simulink model "control_pos_3dof_sinMI"  (R2023b)
settings: Solver=ode5  StartTime=0.0  StopTime=tsim  FixedStep=tstep  RelTol=1e-3
undefined symbols (not defined in the file): a0, a1, robot_params, t_qeq_init, t_tr_init, tau_L
(part 2 of 2)

== matlab function control_pos_3dof_sinMI/Modelo robot manipulador (Dinámica directa)/Modelo dinámico ==
  data: robot_params input; robot_din output Bus: robot_din_bus size=1; q input size=[3,1]; dq input size=[3,1]
function robot_din = fcn(robot_params,q,dq)

%d1 = robot_params.d(1);
l2 = robot_params.l(2);
lc2 = robot_params.lc(2);
%l3 = robot_params.l(3);
lc3 = robot_params.lc(3);

%m1 = robot_params.m(1);
m2 = robot_params.m(2);
m3 = robot_params.m(3);

Iz1 = robot_params.I(1,3);
Iy2 = robot_params.I(2,2);
Iz2 = robot_params.I(2,3);
Iy3 = robot_params.I(3,2);
Iz3 = robot_params.I(3,3);

g = 9.81;

q1 = q(1);
q2 = q(2);
q3 = q(3);

dq1 = dq(1);
dq2 = dq(2);
dq3 = dq(3);

D = zeros(3,3);

D(1,1) = Iz1 + Iz2 + Iz3 + (m2/2)*lc2^2*(1+cos(2*q2)) ...
       + (m3/2)*(l2^2*(1+cos(2*q2)) + 2*l2*lc3*(cos(2*q2+q3)+cos(q3)) ...
       + lc3^2*(1+cos(2*q2+2*q3)));

D(2,2) = Iy2 + Iy3 + m2*lc2^2 + m3*(l2^2 + 2*l2*lc3*cos(q3) + lc3^2);
D(2,3) = Iy3 + m3*(l2*lc3*cos(q3) + lc3^2);

D(3,2) = Iy3 + m3*(l2*lc3*cos(q3) + lc3^2);
D(3,3) = Iy3 + m3*lc3^2;

C = zeros(3,3);

C(1,2) = - ((m2*lc2^2*sin(2*q2)) ...
         + m3*(l2^2*sin(2*q2) + 2*l2*lc3*sin(2*q2+q3) ...
         + lc3^2*sin(2*q2+2*q3)))*dq1;
C(1,3) = - m3*(l2*lc3*(sin(2*q2+q3)+sin(q3)) ...
         + lc3^2*(sin(2*q2+2*q3)))*dq1;

C(2,1) =   ((m2/2)*(lc2^2*sin(2*q2)) ...
         + (m3/2)*(l2^2*sin(2*q2) + 2*l2*lc3*sin(2*q2+q3) ...
         + lc3^2*sin(2*q2+2*q3)))*dq1;
C(2,2) = - 2*m3*l2*lc3*sin(q3)*dq3;
C(2,3) = - m3*l2*lc3*sin(q3)*dq3;

C(3,1) =   (m3/2)*(l2*lc3*(sin(2*q2+q3) + sin(q3)) ...
         + lc3^2*sin(2*q2+2*q3))*dq1;
C(3,2) =   m3*l2*lc3*sin(q3)*dq2;

G = zeros(3,1);

G(2,1) = m2*lc2*cos(q2) + m3*(l2*cos(q2) + lc3*cos(q2+q3));
G(3,1) = m3*lc3*cos(q2+q3);


robot_din = struct('D',D,'C',C,'G',G,'g',9.81);

%busInfo = Simulink.Bus.createObject(robot_dyn);

== matlab function control_pos_3dof_sinMI/q to xyz (robot)/Cinemática directa ==
  data: robot_params input; p output size=[3,3]; q input size=[3,1]
function p  = fcn(robot_params,q)

d1 = robot_params.d(1);
l2 = robot_params.l(2);
l3 = robot_params.l(3);

q1 = q(1);
q2 = q(2);
q3 = q(3);

p1 = [0;0;d1];

p2 = [l2*cos(q1)*cos(q2);
      l2*sin(q1)*cos(q2);
      d1+l2*sin(q2)];

p3 = [cos(q1)*(l2*cos(q2)+l3*cos(q2+q3));
      sin(q1)*(l2*cos(q2)+l3*cos(q2+q3));
      d1+l2*sin(q2)+l3*sin(q2+q3)];

p = [p1,p2,p3];

== matlab function control_pos_3dof_sinMI/q to xyz (referencia)/ddq to ddp ==
  data: dJP input size=[3,3]; ddp output size=[3,1]; ddq input size=[3,1]
function ddp = fcn(dJP,ddq)

ddp = dJP*ddq;

== matlab function control_pos_3dof_sinMI/q to xyz (referencia)/dq to dp ==
  data: JP input size=[3,3]; dp output size=[3,1]; dq input size=[3,1]
function dp = fcn(JP,dq)

dp = JP*dq;

== matlab function control_pos_3dof_sinMI/q to xyz (robot)/Jacobiano ==
  data: robot_params input; JP output size=[3,3]; q input size=[3,1]
function JP = fcn(robot_params,q)

l2 = robot_params.l(2);
l3 = robot_params.l(3);

q1 = q(1);
q2 = q(2);
q3 = q(3);

JP = zeros(3,3);

JP(1,1) = -sin(q1)*(l2*cos(q2) + l3*cos(q2 + q3));
JP(1,2) = -cos(q1)*(l2*sin(q2) + l3*sin(q2 + q3));
JP(1,3) = -l3*cos(q1)*sin(q2 + q3);

JP(2,1) =  cos(q1)*(l2*cos(q2) + l3*cos(q2 + q3));
JP(2,2) = -sin(q1)*(l2*sin(q2) + l3*sin(q2 + q3));
JP(2,3) = -l3*sin(q1)*sin(q2 + q3);

JP(3,2) = l2*cos(q2) + l3*cos(q2 + q3);
JP(3,3) = l3*cos(q2 + q3);

== matlab function control_pos_3dof_sinMI/q to xyz (robot)/ddq to ddp ==
  data: dJP input size=[3,3]; ddp output size=[3,1]; ddq input size=[3,1]
function ddp = fcn(dJP,ddq)

ddp = dJP*ddq;

== matlab function control_pos_3dof_sinMI/q to xyz (robot)/derivada Jacobiano ==
  data: robot_params input; q input size=[3,1]; dJP output size=[3,3]; dq input size=[3,1]
function dJP = dJP(robot_params,q,dq)

l2 = robot_params.l(2);
l3 = robot_params.l(3);

dq1 = dq(1);
dq2 = dq(2);
dq3 = dq(3);


q1 = q(1);
q2 = q(2);
q3 = q(3);

dJP = zeros(3,3);

dJP(1,1) = - cos(q1)*(l2*cos(q2) + l3*cos(q2 + q3))*dq1 + sin(q1)*(l2*sin(q2) + l3*sin(q2 + q3))*dq2 + l3*sin(q1)*sin(q2 + q3)*dq3;
dJP(1,2) =   sin(q1)*(l2*sin(q2) + l3*sin(q2 + q3))*dq1 - cos(q1)*(l2*cos(q2) + l3*cos(q2 + q3))*dq2 - l3*cos(q1)*cos(q2 + q3)*dq3;
dJP(1,3) =   l3*sin(q1)*sin(q2 + q3)*dq1 - l3*cos(q1)*cos(q2 + q3)*dq2 - l3*cos(q1)*cos(q2 + q3)*dq3;

dJP(2,1) = - sin(q1)*(l2*cos(q2) + l3*cos(q2 + q3))*dq1 - cos(q1)*(l2*sin(q2) + l3*sin(q2 + q3))*dq2 - l3*cos(q1)*sin(q2 + q3)*dq3;
dJP(2,2) = - cos(q1)*(l2*sin(q2) + l3*sin(q2 + q3))*dq1 - sin(q1)*(l2*cos(q2) + l3*cos(q2 + q3))*dq2 - l3*sin(q1)*cos(q2 + q3)*dq3;
dJP(2,3) = - l3*cos(q1)*sin(q2 + q3)*dq1 - l3*sin(q1)*cos(q2 + q3)*dq2 - l3*sin(q1)*cos(q2 + q3)*dq3;

dJP(3,1) = 0;
dJP(3,2) = - (l2*sin(q2) + l3*sin(q2 + q3))*dq2 - l3*sin(q2 + q3)*dq3;
dJP(3,3) = - l3*sin(q2 + q3)*(dq2 + dq3);

== matlab function control_pos_3dof_sinMI/Modelo robot manipulador (Dinámica directa)/Dinámica directa ==
  data: robot_din input; ddq output size=[3,1]; dq input size=[3,1]; tau_R input size=[3,1]; tau_L input size=[3,1]
function ddq = fcn(robot_din,dq,tau_R,tau_L)

D = robot_din.D;
C = robot_din.C;
G = robot_din.G;
g = robot_din.g;

ddq = D^-1*(-C*dq-G*g+(tau_R-tau_L));

== matlab function control_pos_3dof_sinMI/xyz to q (referencia)/xyz to q (referencia) ==
  data: robot_params input; q output size=[3,1]; r input size=[3,1]; dr input size=[3,1]; ddr input size=[3,1]; dq output size=[3,1]; ddq output size=[3,1]
function [q,dq,ddq] = fcn(robot_params,r,dr,ddr)

d1 = robot_params.d(1);
l2 = robot_params.l(2);
l3 = robot_params.l(3);

Xr = r(1);
Yr = r(2);
Zr = r(3);


c3 = (Xr^2+Yr^2+(Zr-d1)^2-l2^2-l3^2)/(2*l2*l3);

q1 = atan2(Yr,Xr);
q2 = atan2(Zr-d1,sqrt(Xr^2+Yr^2)) - atan2(-l3*sqrt(1-c3^2),l2+l3*c3);
q3 = atan2(-sqrt(1-c3^2),c3);

q = [q1;q2;q3];

JPinv = zeros(3,3);
JPinv(1,1) = -sin(q1)/(l2*cos(q2) + l3*cos(q2 + q3));
JPinv(1,2) = cos(q1)/(l2*cos(q2) + l3*cos(q2 + q3));

JPinv(2,1) = cos(q1)*cos(q2 + q3)/(l2*sin(q3));
JPinv(2,2) = sin(q1)*cos(q2 + q3)/(l2*sin(q3));
JPinv(2,3) = sin(q2 + q3)/(l2*sin(q3));

JPinv(3,1) = -(cos(q1)*(l2*cos(q2) + l3*cos(q2 + q3)))/(l2*l3*sin(q3));
JPinv(3,2) = -(sin(q1)*(l2*cos(q2) + l3*cos(q2 + q3)))/(l2*l3*sin(q3));
JPinv(3,3) = -(l2*sin(q2) + l3*sin(q2 + q3))/(l2*l3*sin(q3));

dq = JPinv*dr;

dq1 = dq(1);
dq2 = dq(2);
dq3 = dq(3);


dJ = zeros(3,3);

dJ(1,1) = - cos(q1)*(l2*cos(q2) + l3*cos(q2 + q3))*dq1 + sin(q1)*(l2*sin(q2) + l3*sin(q2 + q3))*dq2 + l3*sin(q1)*sin(q2 + q3)*dq3;
dJ(1,2) =   sin(q1)*(l2*sin(q2) + l3*sin(q2 + q3))*dq1 - cos(q1)*(l2*cos(q2) + l3*cos(q2 + q3))*dq2 - l3*cos(q1)*cos(q2 + q3)*dq3;
dJ(1,3) =   l3*sin(q1)*sin(q2 + q3)*dq1 - l3*cos(q1)*cos(q2 + q3)*dq2 - l3*cos(q1)*cos(q2 + q3)*dq3;

dJ(2,1) = - sin(q1)*(l2*cos(q2) + l3*cos(q2 + q3))*dq1 - cos(q1)*(l2*sin(q2) + l3*sin(q2 + q3))*dq2 - l3*cos(q1)*sin(q2 + q3)*dq3;
dJ(2,2) = - cos(q1)*(l2*sin(q2) + l3*sin(q2 + q3))*dq1 - sin(q1)*(l2*cos(q2) + l3*cos(q2 + q3))*dq2 - l3*sin(q1)*cos(q2 + q3)*dq3;
dJ(2,3) = - l3*cos(q1)*sin(q2 + q3)*dq1 - l3*sin(q1)*cos(q2 + q3)*dq2 - l3*sin(q1)*cos(q2 + q3)*dq3;

dJ(3,1) = 0;
dJ(3,2) = - (l2*sin(q2) + l3*sin(q2 + q3))*dq2 - l3*sin(q2 + q3)*dq3;
dJ(3,3) = - l3*sin(q2 + q3)*(dq2 + dq3);

ddq = JPinv*(ddr - dJ*dq);

== matlab function control_pos_3dof_sinMI/q to xyz (robot)/dq to dp ==
  data: JP input size=[3,3]; dp output size=[3,1]; dq input size=[3,1]
function dp = fcn(JP,dq)

dp = JP*dq;

== matlab function control_pos_3dof_sinMI/q to xyz (robot)/q to xyz (referencia) ==
  data: robot_params input; p output size=[3,3]; q input size=[3,1]; dq input size=[3,1]; ddq input size=[3,1]; dp output size=[3,1]; ddp output size=[3,1]
function [p,dp,ddp] = fcn(robot_params,q,dq,ddq)

d1 = robot_params.d(1);
l2 = robot_params.l(2);
l3 = robot_params.l(3);

q1 = q(1);
q2 = q(2);
q3 = q(3);

p1 = [0;0;d1];

p2 = [l2*cos(q1)*cos(q2);
      l2*sin(q1)*cos(q2);
      d1+l2*sin(q2)];

p3 = [cos(q1)*(l2*cos(q2)+l3*cos(q2+q3));
      sin(q1)*(l2*cos(q2)+l3*cos(q2+q3));
      d1+l2*sin(q2)+l3*sin(q2+q3)];

p = [p1,p2,p3];

JP = zeros(3,3);

JP(1,1) = -sin(q1)*(l2*cos(q2) + l3*cos(q2 + q3));
JP(1,2) = -cos(q1)*(l2*sin(q2) + l3*sin(q2 + q3));
JP(1,3) = -l3*cos(q1)*sin(q2 + q3);

JP(2,1) =  cos(q1)*(l2*cos(q2) + l3*cos(q2 + q3));
JP(2,2) = -sin(q1)*(l2*sin(q2) + l3*sin(q2 + q3));
JP(2,3) = -l3*sin(q1)*sin(q2 + q3);

JP(3,2) = l2*cos(q2) + l3*cos(q2 + q3);
JP(3,3) = l3*cos(q2 + q3);

dp = JP*dq;
dq1 = dq(1);
dq2 = dq(2);
dq3 = dq(3);

dJ = zeros(3,3);

dJ(1,1) = - cos(q1)*(l2*cos(q2) + l3*cos(q2 + q3))*dq1 + sin(q1)*(l2*sin(q2) + l3*sin(q2 + q3))*dq2 + l3*sin(q1)*sin(q2 + q3)*dq3;
dJ(1,2) =   sin(q1)*(l2*sin(q2) + l3*sin(q2 + q3))*dq1 - cos(q1)*(l2*cos(q2) + l3*cos(q2 + q3))*dq2 - l3*cos(q1)*cos(q2 + q3)*dq3;
dJ(1,3) =   l3*sin(q1)*sin(q2 + q3)*dq1 - l3*cos(q1)*cos(q2 + q3)*dq2 - l3*cos(q1)*cos(q2 + q3)*dq3;

dJ(2,1) = - sin(q1)*(l2*cos(q2) + l3*cos(q2 + q3))*dq1 - cos(q1)*(l2*sin(q2) + l3*sin(q2 + q3))*dq2 - l3*cos(q1)*sin(q2 + q3)*dq3;
dJ(2,2) = - cos(q1)*(l2*sin(q2) + l3*sin(q2 + q3))*dq1 - sin(q1)*(l2*cos(q2) + l3*cos(q2 + q3))*dq2 - l3*sin(q1)*cos(q2 + q3)*dq3;
dJ(2,3) = - l3*cos(q1)*sin(q2 + q3)*dq1 - l3*sin(q1)*cos(q2 + q3)*dq2 - l3*sin(q1)*cos(q2 + q3)*dq3;

dJ(3,1) = 0;
dJ(3,2) = - (l2*sin(q2) + l3*sin(q2 + q3))*dq2 - l3*sin(q2 + q3)*dq3;
dJ(3,3) = - l3*sin(q2 + q3)*(dq2 + dq3);

ddp = dJ*ddq;

== matlab function control_pos_3dof_sinMI/Controlador/Controlador ==
  data: robot_din input; tau_R output size=[3,1]; A0 input size=[3,1]; A1 input size=[3,1]; q_ref input size=[3,1]; dq_ref input size=[3,1]; ddq_ref input size=[3,1]; q input size=[3,1]; dq input size=[3,1]
function tau_R = fcn(robot_din,A0,A1,q_ref,dq_ref,ddq_ref,q,dq)

D = robot_din.D;
C = robot_din.C;
G = robot_din.G;
g = robot_din.g;

tau_R = D*(ddq_ref+A1.*dq_ref+A0.*q_ref-A1.*dq-A0.*q)+(C*dq+G*g);

== matlab function control_pos_3dof_sinMI/Inicializar posición de robot manipulador/dq_init/q1/Polinomio 7mo orden dq ==
  data: t input; q0 input; qpol output; vpol output; apol output; jpol output; q1 input; t0 input; t1 input
function [qpol,vpol,apol,jpol] = fcn(t,q0,q1,t0,t1)


% t,q0,q1,v0,v1,ac0,ac1,j0,j1,t0,t1)
%Trayectoria de referencia

% q0 = 0;
% q1 = 0;

v0 = 0;
v1 = 0;

ac0 = 0;
ac1 = 0;

j0 = 0;
j1 = 0;

% t0 = 0;
% t1 = pi/4;

% Coeficientes de un polinomio de 7mo grado

h = q1 - q0;
T = t1 - t0;

a = zeros(7+1,1);

a(1) = q0;
a(2) = v0;
a(3) = ac0/2;
a(4) = j0/6;
a(5) = (210*h-T*((30*ac0-15*ac1)*T+(4*j0+j1)*T^2+120*v0+90*v1))/(6*T^4);
a(6) = (-168*h-T*((20*ac0-14*ac1)*T+(2*j0+j1)*T^2+90*v0+78*v1))/(2*T^5);
a(7) = (420*h-T*((45*ac0-39*ac1)*T+(4*j0+3*j1)*T^2+216*v0+204*v1))/(6*T^6);
a(8) = (-120*h-T*((12*ac0-12*ac1)*T+(j0+j1)*T^2+60*v0+60*v1))/(6*T^7);

qa = flip(a')';
va = polyder(qa')';
aa = polyder(va')';
ja = polyder(aa')';


if t>=t0 && t<t1
    qpol = polyval(qa,t-t0);
    vpol = polyval(va,t-t0);
    apol = polyval(aa,t-t0);
    jpol = polyval(ja,t-t0);
elseif t>=t1
    qpol = polyval(qa,T);
    vpol = polyval(va,T);
    apol = polyval(aa,T);
    jpol = polyval(ja,T);
else
    qpol = q0;
    vpol = v0;
    apol = ac0;
    jpol = j0;
end

== matlab function control_pos_3dof_sinMI/Inicializar posición de robot manipulador/dq_init/q2/Polinomio 7mo orden dq ==
  data: t input; q0 input; qpol output; vpol output; apol output; jpol output; q1 input; t0 input; t1 input
function [qpol,vpol,apol,jpol] = fcn(t,q0,q1,t0,t1)


% t,q0,q1,v0,v1,ac0,ac1,j0,j1,t0,t1)
%Trayectoria de referencia

% q0 = 0;
% q1 = 0;

v0 = 0;
v1 = 0;

ac0 = 0;
ac1 = 0;

j0 = 0;
j1 = 0;

% t0 = 0;
% t1 = pi/4;

% Coeficientes de un polinomio de 7mo grado

h = q1 - q0;
T = t1 - t0;

a = zeros(7+1,1);

a(1) = q0;
a(2) = v0;
a(3) = ac0/2;
a(4) = j0/6;
a(5) = (210*h-T*((30*ac0-15*ac1)*T+(4*j0+j1)*T^2+120*v0+90*v1))/(6*T^4);
a(6) = (-168*h-T*((20*ac0-14*ac1)*T+(2*j0+j1)*T^2+90*v0+78*v1))/(2*T^5);
a(7) = (420*h-T*((45*ac0-39*ac1)*T+(4*j0+3*j1)*T^2+216*v0+204*v1))/(6*T^6);
a(8) = (-120*h-T*((12*ac0-12*ac1)*T+(j0+j1)*T^2+60*v0+60*v1))/(6*T^7);

qa = flip(a')';
va = polyder(qa')';
aa = polyder(va')';
ja = polyder(aa')';


if t>=t0 && t<t1
    qpol = polyval(qa,t-t0);
    vpol = polyval(va,t-t0);
    apol = polyval(aa,t-t0);
    jpol = polyval(ja,t-t0);
elseif t>=t1
    qpol = polyval(qa,T);
    vpol = polyval(va,T);
    apol = polyval(aa,T);
    jpol = polyval(ja,T);
else
    qpol = q0;
    vpol = v0;
    apol = ac0;
    jpol = j0;
end

== matlab function control_pos_3dof_sinMI/Inicializar posición de robot manipulador/dq_init/q3/Polinomio 7mo orden dq ==
  data: t input; q0 input; qpol output; vpol output; apol output; jpol output; q1 input; t0 input; t1 input
function [qpol,vpol,apol,jpol] = fcn(t,q0,q1,t0,t1)


% t,q0,q1,v0,v1,ac0,ac1,j0,j1,t0,t1)
%Trayectoria de referencia

% q0 = 0;
% q1 = 0;

v0 = 0;
v1 = 0;

ac0 = 0;
ac1 = 0;

j0 = 0;
j1 = 0;

% t0 = 0;
% t1 = pi/4;

% Coeficientes de un polinomio de 7mo grado

h = q1 - q0;
T = t1 - t0;

a = zeros(7+1,1);

a(1) = q0;
a(2) = v0;
a(3) = ac0/2;
a(4) = j0/6;
a(5) = (210*h-T*((30*ac0-15*ac1)*T+(4*j0+j1)*T^2+120*v0+90*v1))/(6*T^4);
a(6) = (-168*h-T*((20*ac0-14*ac1)*T+(2*j0+j1)*T^2+90*v0+78*v1))/(2*T^5);
a(7) = (420*h-T*((45*ac0-39*ac1)*T+(4*j0+3*j1)*T^2+216*v0+204*v1))/(6*T^6);
a(8) = (-120*h-T*((12*ac0-12*ac1)*T+(j0+j1)*T^2+60*v0+60*v1))/(6*T^7);

qa = flip(a')';
va = polyder(qa')';
aa = polyder(va')';
ja = polyder(aa')';


if t>=t0 && t<t1
    qpol = polyval(qa,t-t0);
    vpol = polyval(va,t-t0);
    apol = polyval(aa,t-t0);
    jpol = polyval(ja,t-t0);
elseif t>=t1
    qpol = polyval(qa,T);
    vpol = polyval(va,T);
    apol = polyval(aa,T);
    jpol = polyval(ja,T);
else
    qpol = q0;
    vpol = v0;
    apol = ac0;
    jpol = j0;
end

== matlab function control_pos_3dof_sinMI/Inicializar posición de robot manipulador/dq_init1/q1/Polinomio 7mo orden dq ==
  data: t input; q0 input; qpol output; vpol output; apol output; jpol output; q1 input; t0 input; t1 input
function [qpol,vpol,apol,jpol] = fcn(t,q0,q1,t0,t1)


% t,q0,q1,v0,v1,ac0,ac1,j0,j1,t0,t1)
%Trayectoria de referencia

% q0 = 0;
% q1 = 0;

v0 = 0;
v1 = 0;

ac0 = 0;
ac1 = 0;

j0 = 0;
j1 = 0;

% t0 = 0;
% t1 = pi/4;

% Coeficientes de un polinomio de 7mo grado

h = q1 - q0;
T = t1 - t0;

a = zeros(7+1,1);

a(1) = q0;
a(2) = v0;
a(3) = ac0/2;
a(4) = j0/6;
a(5) = (210*h-T*((30*ac0-15*ac1)*T+(4*j0+j1)*T^2+120*v0+90*v1))/(6*T^4);
a(6) = (-168*h-T*((20*ac0-14*ac1)*T+(2*j0+j1)*T^2+90*v0+78*v1))/(2*T^5);
a(7) = (420*h-T*((45*ac0-39*ac1)*T+(4*j0+3*j1)*T^2+216*v0+204*v1))/(6*T^6);
a(8) = (-120*h-T*((12*ac0-12*ac1)*T+(j0+j1)*T^2+60*v0+60*v1))/(6*T^7);

qa = flip(a')';
va = polyder(qa')';
aa = polyder(va')';
ja = polyder(aa')';


if t>=t0 && t<t1
    qpol = polyval(qa,t-t0);
    vpol = polyval(va,t-t0);
    apol = polyval(aa,t-t0);
    jpol = polyval(ja,t-t0);
elseif t>=t1
    qpol = polyval(qa,T);
    vpol = polyval(va,T);
    apol = polyval(aa,T);
    jpol = polyval(ja,T);
else
    qpol = q0;
    vpol = v0;
    apol = ac0;
    jpol = j0;
end

== matlab function control_pos_3dof_sinMI/Inicializar posición de robot manipulador/dq_init1/q2/Polinomio 7mo orden dq ==
  data: t input; q0 input; qpol output; vpol output; apol output; jpol output; q1 input; t0 input; t1 input
function [qpol,vpol,apol,jpol] = fcn(t,q0,q1,t0,t1)


% t,q0,q1,v0,v1,ac0,ac1,j0,j1,t0,t1)
%Trayectoria de referencia

% q0 = 0;
% q1 = 0;

v0 = 0;
v1 = 0;

ac0 = 0;
ac1 = 0;

j0 = 0;
j1 = 0;

% t0 = 0;
% t1 = pi/4;

% Coeficientes de un polinomio de 7mo grado

h = q1 - q0;
T = t1 - t0;

a = zeros(7+1,1);

a(1) = q0;
a(2) = v0;
a(3) = ac0/2;
a(4) = j0/6;
a(5) = (210*h-T*((30*ac0-15*ac1)*T+(4*j0+j1)*T^2+120*v0+90*v1))/(6*T^4);
a(6) = (-168*h-T*((20*ac0-14*ac1)*T+(2*j0+j1)*T^2+90*v0+78*v1))/(2*T^5);
a(7) = (420*h-T*((45*ac0-39*ac1)*T+(4*j0+3*j1)*T^2+216*v0+204*v1))/(6*T^6);
a(8) = (-120*h-T*((12*ac0-12*ac1)*T+(j0+j1)*T^2+60*v0+60*v1))/(6*T^7);

qa = flip(a')';
va = polyder(qa')';
aa = polyder(va')';
ja = polyder(aa')';


if t>=t0 && t<t1
    qpol = polyval(qa,t-t0);
    vpol = polyval(va,t-t0);
    apol = polyval(aa,t-t0);
    jpol = polyval(ja,t-t0);
elseif t>=t1
    qpol = polyval(qa,T);
    vpol = polyval(va,T);
    apol = polyval(aa,T);
    jpol = polyval(ja,T);
else
    qpol = q0;
    vpol = v0;
    apol = ac0;
    jpol = j0;
end

== matlab function control_pos_3dof_sinMI/Inicializar posición de robot manipulador/dq_init1/q3/Polinomio 7mo orden dq ==
  data: t input; q0 input; qpol output; vpol output; apol output; jpol output; q1 input; t0 input; t1 input
function [qpol,vpol,apol,jpol] = fcn(t,q0,q1,t0,t1)


% t,q0,q1,v0,v1,ac0,ac1,j0,j1,t0,t1)
%Trayectoria de referencia

% q0 = 0;
% q1 = 0;

v0 = 0;
v1 = 0;

ac0 = 0;
ac1 = 0;

j0 = 0;
j1 = 0;

% t0 = 0;
% t1 = pi/4;

% Coeficientes de un polinomio de 7mo grado

h = q1 - q0;
T = t1 - t0;

a = zeros(7+1,1);

a(1) = q0;
a(2) = v0;
a(3) = ac0/2;
a(4) = j0/6;
a(5) = (210*h-T*((30*ac0-15*ac1)*T+(4*j0+j1)*T^2+120*v0+90*v1))/(6*T^4);
a(6) = (-168*h-T*((20*ac0-14*ac1)*T+(2*j0+j1)*T^2+90*v0+78*v1))/(2*T^5);
a(7) = (420*h-T*((45*ac0-39*ac1)*T+(4*j0+3*j1)*T^2+216*v0+204*v1))/(6*T^6);
a(8) = (-120*h-T*((12*ac0-12*ac1)*T+(j0+j1)*T^2+60*v0+60*v1))/(6*T^7);

qa = flip(a')';
va = polyder(qa')';
aa = polyder(va')';
ja = polyder(aa')';


if t>=t0 && t<t1
    qpol = polyval(qa,t-t0);
    vpol = polyval(va,t-t0);
    apol = polyval(aa,t-t0);
    jpol = polyval(ja,t-t0);
elseif t>=t1
    qpol = polyval(qa,T);
    vpol = polyval(va,T);
    apol = polyval(aa,T);
    jpol = polyval(ja,T);
else
    qpol = q0;
    vpol = v0;
    apol = ac0;
    jpol = j0;
end

== matlab function control_pos_3dof_sinMI/Controlador/Controlador no lineal ==
  data: robot_params input; tau_R output size=[3,1]; q_ref input size=[3,1]; dq_ref input size=[3,1]; ddq_ref input size=[3,1]; q input size=[3,1]; dq input size=[3,1]; A0 input size=[3,1]; A1 input size=[3,1]
function tau_R = fcn(robot_params,q_ref,dq_ref,ddq_ref,q,dq,A0,A1)

%d1 = robot_params.d(1);
l2 = robot_params.l(2);
lc2 = robot_params.lc(2);
%l3 = robot_params.l(3);
lc3 = robot_params.lc(3);

%m1 = robot_params.m(1);
m2 = robot_params.m(2);
m3 = robot_params.m(3);

Iz1 = robot_params.I(1,3);
Iy2 = robot_params.I(2,2);
Iz2 = robot_params.I(2,3);
Iy3 = robot_params.I(3,2);
Iz3 = robot_params.I(3,3);

g = 9.81;

%q1 = q(1);
q2 = q(2);
q3 = q(3);

dq1 = dq(1);
dq2 = dq(2);
dq3 = dq(3);

D = zeros(3,3);

D(1,1) = Iz1 + Iz2 + Iz3 + (m2/2)*lc2^2*(1+cos(2*q2)) ...
       + (m3/2)*(l2^2*(1+cos(2*q2)) + 2*l2*lc3*(cos(2*q2+q3)+cos(q3)) ...
       + lc3^2*(1+cos(2*q2+2*q3)));

D(2,2) = Iy2 + Iy3 + m2*lc2^2 + m3*(l2^2 + 2*l2*lc3*cos(q3) + lc3^2);
D(2,3) = Iy3 + m3*(l2*lc3*cos(q3) + lc3^2);

D(3,2) = Iy3 + m3*(l2*lc3*cos(q3) + lc3^2);
D(3,3) = Iy3 + m3*lc3^2;

C = zeros(3,3);

C(1,2) = - ((m2*lc2^2*sin(2*q2)) ...
         + m3*(l2^2*sin(2*q2) + 2*l2*lc3*sin(2*q2+q3) ...
         + lc3^2*sin(2*q2+2*q3)))*dq1;
C(1,3) = - m3*(l2*lc3*(sin(2*q2+q3)+sin(q3)) ...
         + lc3^2*(sin(2*q2+2*q3)))*dq1;

C(2,1) =   ((m2/2)*(lc2^2*sin(2*q2)) ...
         + (m3/2)*(l2^2*sin(2*q2) + 2*l2*lc3*sin(2*q2+q3) ...
         + lc3^2*sin(2*q2+2*q3)))*dq1;
C(2,2) = - 2*m3*l2*lc3*sin(q3)*dq3;
C(2,3) = - m3*l2*lc3*sin(q3)*dq3;

C(3,1) =   (m3/2)*(l2*lc3*(sin(2*q2+q3) + sin(q3)) ...
         + lc3^2*sin(2*q2+2*q3))*dq1;
C(3,2) =   m3*l2*lc3*sin(q3)*dq2;

G = zeros(3,1);

G(2,1) = m2*lc2*cos(q2) + m3*(l2*cos(q2) + lc3*cos(q2+q3));
G(3,1) = m3*lc3*cos(q2+q3);

tau_R = D*(ddq_ref+A1.*dq_ref+A0.*q_ref-A1.*dq-A0.*q)+(C*dq+G*g);

== matlab function control_pos_3dof_sinMI/Inicializar posición de robot manipulador/q_init_tr/q1/Polinomio 7mo orden dq ==
  data: t input; q0 input; qpol output; vpol output; apol output; jpol output; q1 input; t0 input; t1 input
function [qpol,vpol,apol,jpol] = fcn(t,q0,q1,t0,t1)


% t,q0,q1,v0,v1,ac0,ac1,j0,j1,t0,t1)
%Trayectoria de referencia

% q0 = 0;
% q1 = 0;

v0 = 0;
v1 = 0;

ac0 = 0;
ac1 = 0;

j0 = 0;
j1 = 0;

% t0 = 0;
% t1 = pi/4;

% Coeficientes de un polinomio de 7mo grado

h = q1 - q0;
T = t1 - t0;

a = zeros(7+1,1);

a(1) = q0;
a(2) = v0;
a(3) = ac0/2;
a(4) = j0/6;
a(5) = (210*h-T*((30*ac0-15*ac1)*T+(4*j0+j1)*T^2+120*v0+90*v1))/(6*T^4);
a(6) = (-168*h-T*((20*ac0-14*ac1)*T+(2*j0+j1)*T^2+90*v0+78*v1))/(2*T^5);
a(7) = (420*h-T*((45*ac0-39*ac1)*T+(4*j0+3*j1)*T^2+216*v0+204*v1))/(6*T^6);
a(8) = (-120*h-T*((12*ac0-12*ac1)*T+(j0+j1)*T^2+60*v0+60*v1))/(6*T^7);

qa = flip(a')';
va = polyder(qa')';
aa = polyder(va')';
ja = polyder(aa')';


if t>=t0 && t<t1
    qpol = polyval(qa,t-t0);
    vpol = polyval(va,t-t0);
    apol = polyval(aa,t-t0);
    jpol = polyval(ja,t-t0);
elseif t>=t1
    qpol = polyval(qa,T);
    vpol = polyval(va,T);
    apol = polyval(aa,T);
    jpol = polyval(ja,T);
else
    qpol = q0;
    vpol = v0;
    apol = ac0;
    jpol = j0;
end

== matlab function control_pos_3dof_sinMI/Inicializar posición de robot manipulador/q_init_tr/q2/Polinomio 7mo orden dq ==
  data: t input; q0 input; qpol output; vpol output; apol output; jpol output; q1 input; t0 input; t1 input
function [qpol,vpol,apol,jpol] = fcn(t,q0,q1,t0,t1)


% t,q0,q1,v0,v1,ac0,ac1,j0,j1,t0,t1)
%Trayectoria de referencia

% q0 = 0;
% q1 = 0;

v0 = 0;
v1 = 0;

ac0 = 0;
ac1 = 0;

j0 = 0;
j1 = 0;

% t0 = 0;
% t1 = pi/4;

% Coeficientes de un polinomio de 7mo grado

h = q1 - q0;
T = t1 - t0;

a = zeros(7+1,1);

a(1) = q0;
a(2) = v0;
a(3) = ac0/2;
a(4) = j0/6;
a(5) = (210*h-T*((30*ac0-15*ac1)*T+(4*j0+j1)*T^2+120*v0+90*v1))/(6*T^4);
a(6) = (-168*h-T*((20*ac0-14*ac1)*T+(2*j0+j1)*T^2+90*v0+78*v1))/(2*T^5);
a(7) = (420*h-T*((45*ac0-39*ac1)*T+(4*j0+3*j1)*T^2+216*v0+204*v1))/(6*T^6);
a(8) = (-120*h-T*((12*ac0-12*ac1)*T+(j0+j1)*T^2+60*v0+60*v1))/(6*T^7);

qa = flip(a')';
va = polyder(qa')';
aa = polyder(va')';
ja = polyder(aa')';


if t>=t0 && t<t1
    qpol = polyval(qa,t-t0);
    vpol = polyval(va,t-t0);
    apol = polyval(aa,t-t0);
    jpol = polyval(ja,t-t0);
elseif t>=t1
    qpol = polyval(qa,T);
    vpol = polyval(va,T);
    apol = polyval(aa,T);
    jpol = polyval(ja,T);
else
    qpol = q0;
    vpol = v0;
    apol = ac0;
    jpol = j0;
end

== matlab function control_pos_3dof_sinMI/Inicializar posición de robot manipulador/q_init_tr/q3/Polinomio 7mo orden dq ==
  data: t input; q0 input; qpol output; vpol output; apol output; jpol output; q1 input; t0 input; t1 input
function [qpol,vpol,apol,jpol] = fcn(t,q0,q1,t0,t1)


% t,q0,q1,v0,v1,ac0,ac1,j0,j1,t0,t1)
%Trayectoria de referencia

% q0 = 0;
% q1 = 0;

v0 = 0;
v1 = 0;

ac0 = 0;
ac1 = 0;

j0 = 0;
j1 = 0;

% t0 = 0;
% t1 = pi/4;

% Coeficientes de un polinomio de 7mo grado

h = q1 - q0;
T = t1 - t0;

a = zeros(7+1,1);

a(1) = q0;
a(2) = v0;
a(3) = ac0/2;
a(4) = j0/6;
a(5) = (210*h-T*((30*ac0-15*ac1)*T+(4*j0+j1)*T^2+120*v0+90*v1))/(6*T^4);
a(6) = (-168*h-T*((20*ac0-14*ac1)*T+(2*j0+j1)*T^2+90*v0+78*v1))/(2*T^5);
a(7) = (420*h-T*((45*ac0-39*ac1)*T+(4*j0+3*j1)*T^2+216*v0+204*v1))/(6*T^6);
a(8) = (-120*h-T*((12*ac0-12*ac1)*T+(j0+j1)*T^2+60*v0+60*v1))/(6*T^7);

qa = flip(a')';
va = polyder(qa')';
aa = polyder(va')';
ja = polyder(aa')';


if t>=t0 && t<t1
    qpol = polyval(qa,t-t0);
    vpol = polyval(va,t-t0);
    apol = polyval(aa,t-t0);
    jpol = polyval(ja,t-t0);
elseif t>=t1
    qpol = polyval(qa,T);
    vpol = polyval(va,T);
    apol = polyval(aa,T);
    jpol = polyval(ja,T);
else
    qpol = q0;
    vpol = v0;
    apol = ac0;
    jpol = j0;
end

== matlab function control_pos_3dof_sinMI/Inicializar posición de robot manipulador/q_init/init_q1/Polinomio 7mo orden q0 ==
  data: t input; q0 input; qpol output; vpol output; apol output; jpol output; q1 input; t0 input; t1 input
function [qpol,vpol,apol,jpol] = fcn(t,q0,q1,t0,t1)


% t,q0,q1,v0,v1,ac0,ac1,j0,j1,t0,t1)
%Trayectoria de referencia

% q0 = 0;
% q1 = 0;

v0 = 0;
v1 = 0;

ac0 = 0;
ac1 = 0;

j0 = 0;
j1 = 0;

% t0 = 0;
% t1 = pi/4;

% Coeficientes de un polinomio de 7mo grado

h = q1 - q0;
T = t1 - t0;

a = zeros(7+1,1);

a(1) = q0;
a(2) = v0;
a(3) = ac0/2;
a(4) = j0/6;
a(5) = (210*h-T*((30*ac0-15*ac1)*T+(4*j0+j1)*T^2+120*v0+90*v1))/(6*T^4);
a(6) = (-168*h-T*((20*ac0-14*ac1)*T+(2*j0+j1)*T^2+90*v0+78*v1))/(2*T^5);
a(7) = (420*h-T*((45*ac0-39*ac1)*T+(4*j0+3*j1)*T^2+216*v0+204*v1))/(6*T^6);
a(8) = (-120*h-T*((12*ac0-12*ac1)*T+(j0+j1)*T^2+60*v0+60*v1))/(6*T^7);

qa = flip(a')';
va = polyder(qa')';
aa = polyder(va')';
ja = polyder(aa')';


if t>=t0 && t<t1
    qpol = polyval(qa,t-t0);
    vpol = polyval(va,t-t0);
    apol = polyval(aa,t-t0);
    jpol = polyval(ja,t-t0);
elseif t>=t1
    qpol = polyval(qa,T);
    vpol = polyval(va,T);
    apol = polyval(aa,T);
    jpol = polyval(ja,T);
else
    qpol = q0;
    vpol = v0;
    apol = ac0;
    jpol = j0;
end

== matlab function control_pos_3dof_sinMI/Inicializar posición de robot manipulador/q_init/init_q1/Polinomio 7mo orden q1 ==
  data: t input; q0 input; qpol output; vpol output; apol output; jpol output; q1 input; t0 input; t1 input
function [qpol,vpol,apol,jpol] = fcn(t,q0,q1,t0,t1)


% t,q0,q1,v0,v1,ac0,ac1,j0,j1,t0,t1)
%Trayectoria de referencia

% q0 = 0;
% q1 = 0;

v0 = 0;
v1 = 0;

ac0 = 0;
ac1 = 0;

j0 = 0;
j1 = 0;

% t0 = 0;
% t1 = pi/4;

% Coeficientes de un polinomio de 7mo grado

h = q1 - q0;
T = t1 - t0;

a = zeros(7+1,1);

a(1) = q0;
a(2) = v0;
a(3) = ac0/2;
a(4) = j0/6;
a(5) = (210*h-T*((30*ac0-15*ac1)*T+(4*j0+j1)*T^2+120*v0+90*v1))/(6*T^4);
a(6) = (-168*h-T*((20*ac0-14*ac1)*T+(2*j0+j1)*T^2+90*v0+78*v1))/(2*T^5);
a(7) = (420*h-T*((45*ac0-39*ac1)*T+(4*j0+3*j1)*T^2+216*v0+204*v1))/(6*T^6);
a(8) = (-120*h-T*((12*ac0-12*ac1)*T+(j0+j1)*T^2+60*v0+60*v1))/(6*T^7);

qa = flip(a')';
va = polyder(qa')';
aa = polyder(va')';
ja = polyder(aa')';


if t>=t0 && t<t1
    qpol = polyval(qa,t-t0);
    vpol = polyval(va,t-t0);
    apol = polyval(aa,t-t0);
    jpol = polyval(ja,t-t0);
elseif t>=t1
    qpol = polyval(qa,T);
    vpol = polyval(va,T);
    apol = polyval(aa,T);
    jpol = polyval(ja,T);
else
    qpol = 0;
    vpol = 0;
    apol = 0;
    jpol = 0;
end

== matlab function control_pos_3dof_sinMI/Inicializar posición de robot manipulador/q_init/init_q2/Polinomio 7mo orden q0 ==
  data: t input; q0 input; qpol output; vpol output; apol output; jpol output; q1 input; t0 input; t1 input
function [qpol,vpol,apol,jpol] = fcn(t,q0,q1,t0,t1)


% t,q0,q1,v0,v1,ac0,ac1,j0,j1,t0,t1)
%Trayectoria de referencia

% q0 = 0;
% q1 = 0;

v0 = 0;
v1 = 0;

ac0 = 0;
ac1 = 0;

j0 = 0;
j1 = 0;

% t0 = 0;
% t1 = pi/4;

% Coeficientes de un polinomio de 7mo grado

h = q1 - q0;
T = t1 - t0;

a = zeros(7+1,1);

a(1) = q0;
a(2) = v0;
a(3) = ac0/2;
a(4) = j0/6;
a(5) = (210*h-T*((30*ac0-15*ac1)*T+(4*j0+j1)*T^2+120*v0+90*v1))/(6*T^4);
a(6) = (-168*h-T*((20*ac0-14*ac1)*T+(2*j0+j1)*T^2+90*v0+78*v1))/(2*T^5);
a(7) = (420*h-T*((45*ac0-39*ac1)*T+(4*j0+3*j1)*T^2+216*v0+204*v1))/(6*T^6);
a(8) = (-120*h-T*((12*ac0-12*ac1)*T+(j0+j1)*T^2+60*v0+60*v1))/(6*T^7);

qa = flip(a')';
va = polyder(qa')';
aa = polyder(va')';
ja = polyder(aa')';


if t>=t0 && t<t1
    qpol = polyval(qa,t-t0);
    vpol = polyval(va,t-t0);
    apol = polyval(aa,t-t0);
    jpol = polyval(ja,t-t0);
elseif t>=t1
    qpol = polyval(qa,T);
    vpol = polyval(va,T);
    apol = polyval(aa,T);
    jpol = polyval(ja,T);
else
    qpol = q0;
    vpol = v0;
    apol = ac0;
    jpol = j0;
end

== matlab function control_pos_3dof_sinMI/Inicializar posición de robot manipulador/q_init/init_q2/Polinomio 7mo orden q1 ==
  data: t input; q0 input; qpol output; vpol output; apol output; jpol output; q1 input; t0 input; t1 input
function [qpol,vpol,apol,jpol] = fcn(t,q0,q1,t0,t1)


% t,q0,q1,v0,v1,ac0,ac1,j0,j1,t0,t1)
%Trayectoria de referencia

% q0 = 0;
% q1 = 0;

v0 = 0;
v1 = 0;

ac0 = 0;
ac1 = 0;

j0 = 0;
j1 = 0;

% t0 = 0;
% t1 = pi/4;

% Coeficientes de un polinomio de 7mo grado

h = q1 - q0;
T = t1 - t0;

a = zeros(7+1,1);

a(1) = q0;
a(2) = v0;
a(3) = ac0/2;
a(4) = j0/6;
a(5) = (210*h-T*((30*ac0-15*ac1)*T+(4*j0+j1)*T^2+120*v0+90*v1))/(6*T^4);
a(6) = (-168*h-T*((20*ac0-14*ac1)*T+(2*j0+j1)*T^2+90*v0+78*v1))/(2*T^5);
a(7) = (420*h-T*((45*ac0-39*ac1)*T+(4*j0+3*j1)*T^2+216*v0+204*v1))/(6*T^6);
a(8) = (-120*h-T*((12*ac0-12*ac1)*T+(j0+j1)*T^2+60*v0+60*v1))/(6*T^7);

qa = flip(a')';
va = polyder(qa')';
aa = polyder(va')';
ja = polyder(aa')';


if t>=t0 && t<t1
    qpol = polyval(qa,t-t0);
    vpol = polyval(va,t-t0);
    apol = polyval(aa,t-t0);
    jpol = polyval(ja,t-t0);
elseif t>=t1
    qpol = polyval(qa,T);
    vpol = polyval(va,T);
    apol = polyval(aa,T);
    jpol = polyval(ja,T);
else
    qpol = 0;
    vpol = 0;
    apol = 0;
    jpol = 0;
end

== matlab function control_pos_3dof_sinMI/Inicializar posición de robot manipulador/q_init/init_q3/Polinomio 7mo orden q0 ==
  data: t input; q0 input; qpol output; vpol output; apol output; jpol output; q1 input; t0 input; t1 input
function [qpol,vpol,apol,jpol] = fcn(t,q0,q1,t0,t1)


% t,q0,q1,v0,v1,ac0,ac1,j0,j1,t0,t1)
%Trayectoria de referencia

% q0 = 0;
% q1 = 0;

v0 = 0;
v1 = 0;

ac0 = 0;
ac1 = 0;

j0 = 0;
j1 = 0;

% t0 = 0;
% t1 = pi/4;

% Coeficientes de un polinomio de 7mo grado

h = q1 - q0;
T = t1 - t0;

a = zeros(7+1,1);

a(1) = q0;
a(2) = v0;
a(3) = ac0/2;
a(4) = j0/6;
a(5) = (210*h-T*((30*ac0-15*ac1)*T+(4*j0+j1)*T^2+120*v0+90*v1))/(6*T^4);
a(6) = (-168*h-T*((20*ac0-14*ac1)*T+(2*j0+j1)*T^2+90*v0+78*v1))/(2*T^5);
a(7) = (420*h-T*((45*ac0-39*ac1)*T+(4*j0+3*j1)*T^2+216*v0+204*v1))/(6*T^6);
a(8) = (-120*h-T*((12*ac0-12*ac1)*T+(j0+j1)*T^2+60*v0+60*v1))/(6*T^7);

qa = flip(a')';
va = polyder(qa')';
aa = polyder(va')';
ja = polyder(aa')';


if t>=t0 && t<t1
    qpol = polyval(qa,t-t0);
    vpol = polyval(va,t-t0);
    apol = polyval(aa,t-t0);
    jpol = polyval(ja,t-t0);
elseif t>=t1
    qpol = polyval(qa,T);
    vpol = polyval(va,T);
    apol = polyval(aa,T);
    jpol = polyval(ja,T);
else
    qpol = q0;
    vpol = v0;
    apol = ac0;
    jpol = j0;
end

== matlab function control_pos_3dof_sinMI/Inicializar posición de robot manipulador/q_init/init_q3/Polinomio 7mo orden q1 ==
  data: t input; q0 input; qpol output; vpol output; apol output; jpol output; q1 input; t0 input; t1 input
function [qpol,vpol,apol,jpol] = fcn(t,q0,q1,t0,t1)


% t,q0,q1,v0,v1,ac0,ac1,j0,j1,t0,t1)
%Trayectoria de referencia

% q0 = 0;
% q1 = 0;

v0 = 0;
v1 = 0;

ac0 = 0;
ac1 = 0;

j0 = 0;
j1 = 0;

% t0 = 0;
% t1 = pi/4;

% Coeficientes de un polinomio de 7mo grado

h = q1 - q0;
T = t1 - t0;

a = zeros(7+1,1);

a(1) = q0;
a(2) = v0;
a(3) = ac0/2;
a(4) = j0/6;
a(5) = (210*h-T*((30*ac0-15*ac1)*T+(4*j0+j1)*T^2+120*v0+90*v1))/(6*T^4);
a(6) = (-168*h-T*((20*ac0-14*ac1)*T+(2*j0+j1)*T^2+90*v0+78*v1))/(2*T^5);
a(7) = (420*h-T*((45*ac0-39*ac1)*T+(4*j0+3*j1)*T^2+216*v0+204*v1))/(6*T^6);
a(8) = (-120*h-T*((12*ac0-12*ac1)*T+(j0+j1)*T^2+60*v0+60*v1))/(6*T^7);

qa = flip(a')';
va = polyder(qa')';
aa = polyder(va')';
ja = polyder(aa')';


if t>=t0 && t<t1
    qpol = polyval(qa,t-t0);
    vpol = polyval(va,t-t0);
    apol = polyval(aa,t-t0);
    jpol = polyval(ja,t-t0);
elseif t>=t1
    qpol = polyval(qa,T);
    vpol = polyval(va,T);
    apol = polyval(aa,T);
    jpol = polyval(ja,T);
else
    qpol = 0;
    vpol = 0;
    apol = 0;
    jpol = 0;
end

== matlab function control_pos_3dof_sinMI/Inicializar posición de robot manipulador/MATLAB Function ==
  data: t input size=1; qi output size=[3,1]; t_init input size=1; q input size=[3,1]; q_init input
function qi  = fcn(t,t_init,q,q_init)

% qi = q;
if t <= t_init
    qi = q;
else
    qi = q_init;
end

== matlab function control_pos_3dof_sinMI/q to xyz (referencia)/q to xyz (referencia) ==
  data: robot_params input; p output size=[3,3]; q input size=[3,1]; dq input size=[3,1]; ddq input size=[3,1]; dp output size=[3,1]; ddp output size=[3,1]
function [p,dp,ddp] = fcn(robot_params,q,dq,ddq)

d1 = robot_params.d(1);
l2 = robot_params.l(2);
l3 = robot_params.l(3);

q1 = q(1);
q2 = q(2);
q3 = q(3);

p1 = [0;0;d1];

p2 = [l2*cos(q1)*cos(q2);
      l2*sin(q1)*cos(q2);
      d1+l2*sin(q2)];

p3 = [cos(q1)*(l2*cos(q2)+l3*cos(q2+q3));
      sin(q1)*(l2*cos(q2)+l3*cos(q2+q3));
      d1+l2*sin(q2)+l3*sin(q2+q3)];

p = [p1,p2,p3];

JP = zeros(3,3);

JP(1,1) = -sin(q1)*(l2*cos(q2) + l3*cos(q2 + q3));
JP(1,2) = -cos(q1)*(l2*sin(q2) + l3*sin(q2 + q3));
JP(1,3) = -l3*cos(q1)*sin(q2 + q3);

JP(2,1) =  cos(q1)*(l2*cos(q2) + l3*cos(q2 + q3));
JP(2,2) = -sin(q1)*(l2*sin(q2) + l3*sin(q2 + q3));
JP(2,3) = -l3*sin(q1)*sin(q2 + q3);

JP(3,2) = l2*cos(q2) + l3*cos(q2 + q3);
JP(3,3) = l3*cos(q2 + q3);

dp = JP*dq;
dq1 = dq(1);
dq2 = dq(2);
dq3 = dq(3);

dJ = zeros(3,3);

dJ(1,1) = - cos(q1)*(l2*cos(q2) + l3*cos(q2 + q3))*dq1 + sin(q1)*(l2*sin(q2) + l3*sin(q2 + q3))*dq2 + l3*sin(q1)*sin(q2 + q3)*dq3;
dJ(1,2) =   sin(q1)*(l2*sin(q2) + l3*sin(q2 + q3))*dq1 - cos(q1)*(l2*cos(q2) + l3*cos(q2 + q3))*dq2 - l3*cos(q1)*cos(q2 + q3)*dq3;
dJ(1,3) =   l3*sin(q1)*sin(q2 + q3)*dq1 - l3*cos(q1)*cos(q2 + q3)*dq2 - l3*cos(q1)*cos(q2 + q3)*dq3;

dJ(2,1) = - sin(q1)*(l2*cos(q2) + l3*cos(q2 + q3))*dq1 - cos(q1)*(l2*sin(q2) + l3*sin(q2 + q3))*dq2 - l3*cos(q1)*sin(q2 + q3)*dq3;
dJ(2,2) = - cos(q1)*(l2*sin(q2) + l3*sin(q2 + q3))*dq1 - sin(q1)*(l2*cos(q2) + l3*cos(q2 + q3))*dq2 - l3*sin(q1)*cos(q2 + q3)*dq3;
dJ(2,3) = - l3*cos(q1)*sin(q2 + q3)*dq1 - l3*sin(q1)*cos(q2 + q3)*dq2 - l3*sin(q1)*cos(q2 + q3)*dq3;

dJ(3,1) = 0;
dJ(3,2) = - (l2*sin(q2) + l3*sin(q2 + q3))*dq2 - l3*sin(q2 + q3)*dq3;
dJ(3,3) = - l3*sin(q2 + q3)*(dq2 + dq3);

ddp = dJ*ddq;

== matlab function control_pos_3dof_sinMI/Controlador/Modelo dinámico ==
  data: robot_params input; robot_din output Bus: robot_din_bus size=1; q input size=[3,1]; dq input size=[3,1]
function robot_din = fcn(robot_params,q,dq)

%d1 = robot_params.d(1);
l2 = robot_params.l(2);
lc2 = robot_params.lc(2);
%l3 = robot_params.l(3);
lc3 = robot_params.lc(3);

%m1 = robot_params.m(1);
m2 = robot_params.m(2);
m3 = robot_params.m(3);

Iz1 = robot_params.I(1,3);
Iy2 = robot_params.I(2,2);
Iz2 = robot_params.I(2,3);
Iy3 = robot_params.I(3,2);
Iz3 = robot_params.I(3,3);

g = 9.81;

q1 = q(1);
q2 = q(2);
q3 = q(3);

dq1 = dq(1);
dq2 = dq(2);
dq3 = dq(3);

D = zeros(3,3);

D(1,1) = Iz1 + Iz2 + Iz3 + (m2/2)*lc2^2*(1+cos(2*q2)) ...
       + (m3/2)*(l2^2*(1+cos(2*q2)) + 2*l2*lc3*(cos(2*q2+q3)+cos(q3)) ...
       + lc3^2*(1+cos(2*q2+2*q3)));

D(2,2) = Iy2 + Iy3 + m2*lc2^2 + m3*(l2^2 + 2*l2*lc3*cos(q3) + lc3^2);
D(2,3) = Iy3 + m3*(l2*lc3*cos(q3) + lc3^2);

D(3,2) = Iy3 + m3*(l2*lc3*cos(q3) + lc3^2);
D(3,3) = Iy3 + m3*lc3^2;

C = zeros(3,3);

C(1,2) = - ((m2*lc2^2*sin(2*q2)) ...
         + m3*(l2^2*sin(2*q2) + 2*l2*lc3*sin(2*q2+q3) ...
         + lc3^2*sin(2*q2+2*q3)))*dq1;
C(1,3) = - m3*(l2*lc3*(sin(2*q2+q3)+sin(q3)) ...
         + lc3^2*(sin(2*q2+2*q3)))*dq1;

C(2,1) =   ((m2/2)*(lc2^2*sin(2*q2)) ...
         + (m3/2)*(l2^2*sin(2*q2) + 2*l2*lc3*sin(2*q2+q3) ...
         + lc3^2*sin(2*q2+2*q3)))*dq1;
C(2,2) = - 2*m3*l2*lc3*sin(q3)*dq3;
C(2,3) = - m3*l2*lc3*sin(q3)*dq3;

C(3,1) =   (m3/2)*(l2*lc3*(sin(2*q2+q3) + sin(q3)) ...
         + lc3^2*sin(2*q2+2*q3))*dq1;
C(3,2) =   m3*l2*lc3*sin(q3)*dq2;

G = zeros(3,1);

G(2,1) = m2*lc2*cos(q2) + m3*(l2*cos(q2) + lc3*cos(q2+q3));
G(3,1) = m3*lc3*cos(q2+q3);


robot_din = struct('D',D,'C',C,'G',G,'g',9.81);

%busInfo = Simulink.Bus.createObject(robot_dyn);

== matlab function control_pos_3dof_sinMI/Dinámica inversa (referencia)/Dinamica inversa (referencia) ==
  data: robot_params input; q input size=[3,1]; tau_s output size=[3,1]; dq input size=[3,1]; ddq input size=[3,1]
function tau_s = dyn_inv(robot_params,q,dq,ddq)

%d1 = robot_params.d(1);
l2 = robot_params.l(2);
lc2 = robot_params.lc(2);
%l3 = robot_params.l(3);
lc3 = robot_params.lc(3);

%m1 = robot_params.m(1);
m2 = robot_params.m(2);
m3 = robot_params.m(3);

Iz1 = robot_params.I(1,3);
Iy2 = robot_params.I(2,2);
Iz2 = robot_params.I(2,3);
Iy3 = robot_params.I(3,2);
Iz3 = robot_params.I(3,3);

g = 9.81;

q1 = q(1);
q2 = q(2);
q3 = q(3);

dq1 = dq(1);
dq2 = dq(2);
dq3 = dq(3);

D = zeros(3,3);

D(1,1) = Iz1 + Iz2 + Iz3 + (m2/2)*lc2^2*(1+cos(2*q2)) ...
       + (m3/2)*(l2^2*(1+cos(2*q2)) + 2*l2*lc3*(cos(2*q2+q3)+cos(q3)) ...
       + lc3^2*(1+cos(2*q2+2*q3)));

D(2,2) = Iy2 + Iy3 + m2*lc2^2 + m3*(l2^2 + 2*l2*lc3*cos(q3) + lc3^2);
D(2,3) = Iy3 + m3*(l2*lc3*cos(q3) + lc3^2);

D(3,2) = Iy3 + m3*(l2*lc3*cos(q3) + lc3^2);
D(3,3) = Iy3 + m3*lc3^2;

C = zeros(3,3);

C(1,2) = - ((m2*lc2^2*sin(2*q2)) ...
         + m3*(l2^2*sin(2*q2) + 2*l2*lc3*sin(2*q2+q3) ...
         + lc3^2*sin(2*q2+2*q3)))*dq1;
C(1,3) = - m3*(l2*lc3*(sin(2*q2+q3)+sin(q3)) ...
         + lc3^2*(sin(2*q2+2*q3)))*dq1;

C(2,1) =   ((m2/2)*(lc2^2*sin(2*q2)) ...
         + (m3/2)*(l2^2*sin(2*q2) + 2*l2*lc3*sin(2*q2+q3) ...
         + lc3^2*sin(2*q2+2*q3)))*dq1;
C(2,2) = - 2*m3*l2*lc3*sin(q3)*dq3;
C(2,3) = - m3*l2*lc3*sin(q3)*dq3;

C(3,1) =   (m3/2)*(l2*lc3*(sin(2*q2+q3) + sin(q3)) ...
         + lc3^2*sin(2*q2+2*q3))*dq1;
C(3,2) =   m3*l2*lc3*sin(q3)*dq2;

G = zeros(3,1);

G(2,1) = m2*lc2*cos(q2) + m3*(l2*cos(q2) + lc3*cos(q2+q3));
G(3,1) = m3*lc3*cos(q2+q3);


tau_s = D*ddq + C*dq + G*g;

== matlab function control_pos_3dof_sinMI/Modelo robot manipulador (Dinámica directa)/Dinámica directa(1) ==
  data: robot_params input; q input size=[3,1]; ddq output size=[3,1]; dq input size=[3,1]; tau_R input size=[3,1]; tau_L input size=[3,1]
function ddq = fcn(robot_params,q,dq,tau_R,tau_L)

%d1 = robot_params.d(1);
l2 = robot_params.l(2);
lc2 = robot_params.lc(2);
%l3 = robot_params.l(3);
lc3 = robot_params.lc(3);

%m1 = robot_params.m(1);
m2 = robot_params.m(2);
m3 = robot_params.m(3);

Iz1 = robot_params.I(1,3);
Iy2 = robot_params.I(2,2);
Iz2 = robot_params.I(2,3);
Iy3 = robot_params.I(3,2);
Iz3 = robot_params.I(3,3);

g = 9.81;

q1 = q(1);
q2 = q(2);
q3 = q(3);

dq1 = dq(1);
dq2 = dq(2);
dq3 = dq(3);

D = zeros(3,3);

D(1,1) = Iz1 + Iz2 + Iz3 + (m2/2)*lc2^2*(1+cos(2*q2)) ...
       + (m3/2)*(l2^2*(1+cos(2*q2)) + 2*l2*lc3*(cos(2*q2+q3)+cos(q3)) ...
       + lc3^2*(1+cos(2*q2+2*q3)));

D(2,2) = Iy2 + Iy3 + m2*lc2^2 + m3*(l2^2 + 2*l2*lc3*cos(q3) + lc3^2);
D(2,3) = Iy3 + m3*(l2*lc3*cos(q3) + lc3^2);

D(3,2) = Iy3 + m3*(l2*lc3*cos(q3) + lc3^2);
D(3,3) = Iy3 + m3*lc3^2;

C = zeros(3,3);

C(1,2) = - ((m2*lc2^2*sin(2*q2)) ...
         + m3*(l2^2*sin(2*q2) + 2*l2*lc3*sin(2*q2+q3) ...
         + lc3^2*sin(2*q2+2*q3)))*dq1;
C(1,3) = - m3*(l2*lc3*(sin(2*q2+q3)+sin(q3)) ...
         + lc3^2*(sin(2*q2+2*q3)))*dq1;

C(2,1) =   ((m2/2)*(lc2^2*sin(2*q2)) ...
         + (m3/2)*(l2^2*sin(2*q2) + 2*l2*lc3*sin(2*q2+q3) ...
         + lc3^2*sin(2*q2+2*q3)))*dq1;
C(2,2) = - 2*m3*l2*lc3*sin(q3)*dq3;
C(2,3) = - m3*l2*lc3*sin(q3)*dq3;

C(3,1) =   (m3/2)*(l2*lc3*(sin(2*q2+q3) + sin(q3)) ...
         + lc3^2*sin(2*q2+2*q3))*dq1;
C(3,2) =   m3*l2*lc3*sin(q3)*dq2;

G = zeros(3,1);

G(2,1) = m2*lc2*cos(q2) + m3*(l2*cos(q2) + lc3*cos(q2+q3));
G(3,1) = m3*lc3*cos(q2+q3);



ddq = D^-1*(-C*dq-G*g+(tau_R-tau_L));

== matlab function control_pos_3dof_sinMI/xyz to q (referencia)/Cinemática inversa ==
  data: robot_params input; q output size=[3,1]; r input size=[3,1]
function q = fcn(robot_params,r)

d1 = robot_params.d(1);
l2 = robot_params.l(2);
l3 = robot_params.l(3);

Xr = r(1);
Yr = r(2);
Zr = r(3);

% Cinematica inversa %%%%%%%%%%%%%%%%%%%%%%%%%%%%%%%%%%%%%%%%%%%%%%%%%%%%%%

c3 = (Xr^2+Yr^2+(Zr-d1)^2-l2^2-l3^2)/(2*l2*l3);

q1 = atan2(Yr,Xr);
q2 = atan2(Zr-d1,sqrt(Xr^2+Yr^2)) - atan2(-l3*sqrt(1-c3^2),l2+l3*c3);
q3 = atan2(-sqrt(1-c3^2),c3);

q = [q1;q2;q3];
